simulink model "model1v3"  (R2020b)
settings: Solver=VariableStepAuto  StartTime=0.0  StopTime=30.0  RelTol=1e-3
settings Model: Creator=dkravchenko  LastModifiedBy=dkravchenko

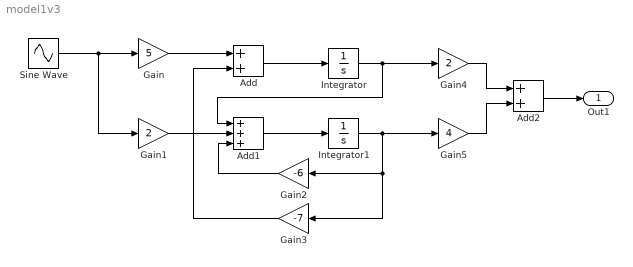
== system model1v3 ==
  Add : Sum
  Add1 : Sum  Inputs=+++
  Add2 : Sum
  Gain : Gain  Gain=5
  Gain1 : Gain  Gain=2
  Gain2 : Gain  Gain=-6
  Gain3 : Gain  Gain=-7
  Gain4 : Gain  Gain=2
  Gain5 : Gain  Gain=4
  Integrator : Integrator  InitialCondition=2
  Integrator1 : Integrator  InitialCondition=0.7
  Sine Wave : Sin  Amplitude=0  SampleTime=0
  Out1 : Outport
  wires:
  Sine Wave/1 -> Gain1/1, Gain/1
  Gain/1 -> Add/1
  Add/1 -> Integrator/1
  Add1/1 -> Integrator1/1
  Gain1/1 -> Add1/2
  Integrator/1 -> Gain4/1, Add1/1
  Integrator1/1 -> Gain3/1, Gain2/1, Gain5/1
  Gain2/1 -> Add1/3
  Gain3/1 -> Add/2
  Gain4/1 -> Add2/1
  Gain5/1 -> Add2/2
  Add2/1 -> Out1/1
